simulink model "TF_simulink"  (R2025a)
settings: Solver=VariableStepAuto  StartTime=0.0  StopTime=50  RelTol=1e-3
undefined symbols (not defined in the file): b, bd, J, Jd, Jmotor, k, kd, ksea
libraries: slpidlib x2
settings Model: Creator=oskar  LastModifiedBy=oskar

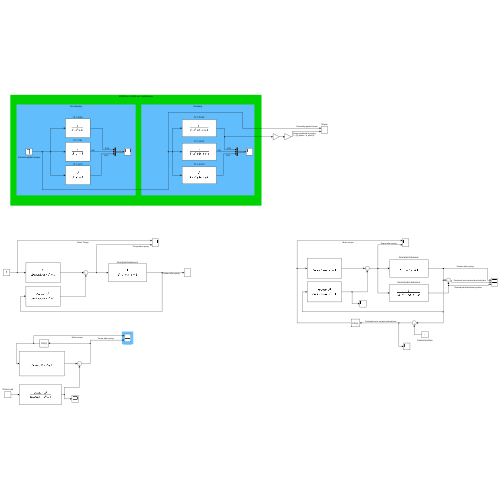
[thumbnail: Simulink's stored preview of the top-level diagram]
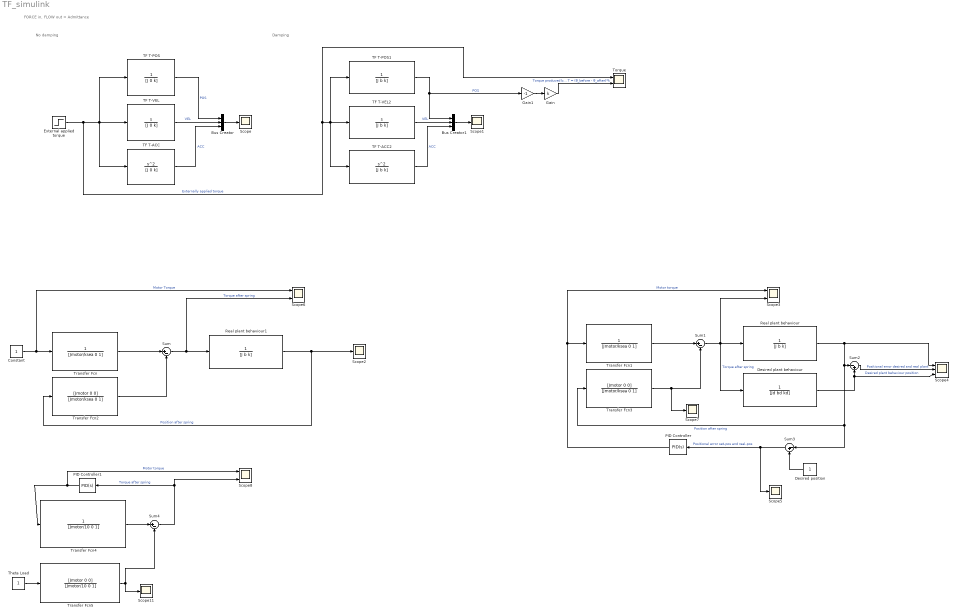
== system TF_simulink ==
  note: FORCE in, FLOW out = Admittance
  note: No damping
  note: Damping
  Bus Creator : BusCreator  Inputs=3
  Bus Creator1 : BusCreator  Inputs=3
  Constant : Constant
  Desired plant behaviour : TransferFcn  Denominator=[Jd bd kd]
  Desired position : Constant
  External applied torque : Step  Time=30  Before=1  After=0  SampleTime=0
  Gain : Gain  Gain=k
  Gain1 : Gain  Gain=-1
  PID Controller : slpidlib/PID Controller  Controller=PID  Form=Parallel  TimeDomain=Continuous-time  UseExternalTs=off  SampleTime=-1  IntegratorMethod=Forward Euler  FilterMethod=Forward Euler  ControllerParametersSource=internal  P=5  I=2  UseKiTs=off  D=0.01  UseExternalDerivativeSource=off  N=100  UseFilter=on  TunerSelectOption=Transfer Function Based (PID Tuner App)  InitialConditionSource=internal  InitialConditionForIntegrator=0  InitialConditionForFilter=0  DifferentiatorICPrevScaledInput=0  ExternalReset=none  TrackingMode=off  Kt=1  LimitOutput=off  SatLimitsSource=internal  UpperSaturationLimit=inf  LowerSaturationLimit=-inf  LinearizeAsGain=on  AntiWindupMode=none  Kb=1  LimitIntegrator=off  UpperIntegratorSaturationLimit=inf  LowerIntegratorSaturationLimit=-inf  POutMin=[]  POutMax=[]  IOutMin=[]  IOutMax=[]  DOutMin=[]  DOutMax=[]  NOutMin=[]  NOutMax=[]  SumOutMin=[]  SumOutMax=[]  SaturationOutMin=[]  SaturationOutMax=[]  PParamMin=[]  PParamMax=[]  IParamMin=[]  IParamMax=[]  DParamMin=[]  DParamMax=[]  NParamMin=[]  NParamMax=[]  KbParamMin=[]  KbParamMax=[]  KtParamMin=[]  KtParamMax=[]  KbOutMin=[]  KbOutMax=[]  KtOutMin=[]  KtOutMax=[]  IntegratorOutMin=[]  IntegratorOutMax=[]  FilterOutMin=[]  FilterOutMax=[]  SumI1OutMin=[]  SumI1OutMax=[]  SumI2OutMin=[]  SumI2OutMax=[]  SumI3OutMin=[]  SumI3OutMax=[]  SumI4OutMin=[]  SumI4OutMax=[]  SumDOutMin=[]  SumDOutMax=[]  DifferentiatorOutMin=[]  DifferentiatorOutMax=[]  FilterDiffOutCoefMin=[]  FilterDiffOutCoefMax=[]  ReciprocalOutMin=[]  ReciprocalOutMax=[]  SumDenOutMin=[]  SumDenOutMax=[]  SumNumOutMin=[]  SumNumOutMax=[]  DivideOutMin=[]  DivideOutMax=[]  UdiffTsProdOutMin=[]  UdiffTsProdOutMax=[]  NTsProdOutMin=[]  NTsProdOutMax=[]  UintegralTsProdOutMin=[]  UintegralTsProdOutMax=[]  UngainTsProdOutMin=[]  UngainTsProdOutMax=[]  ClampingZeroOutDataTypeStr=Inherit: Inherit via back propagation  ClampingZeroOutMin=[]  ClampingZeroOutMax=[]  FilterDenConstantOutDataTypeStr=Inherit: Inherit via back propagation  FilterDenConstantOutMin=[]  FilterDenConstantOutMax=[]  PCopyOutDataTypeStr=Inherit: Inherit via back propagation  PCopyOutMin=[]  PCopyOutMax=[]  NCopyOutDataTypeStr=Inherit: Inherit via back propagation  NCopyOutMin=[]  NCopyOutMax=[]  IntegratorContinuousStateAttributes=''  IntegratorStateMustResolveToSignalObject=off  IntegratorRTWStateStorageClass=Auto  FilterContinuousStateAttributes=''  FilterStateMustResolveToSignalObject=off  FilterRTWStateStorageClass=Auto  ParallelPVariant=InternalParameters  IdealPVariant=Disabled  IVariant=InternalParameters  DVariant=InternalParameters  IntegratorVariant=Continuous  SatVariant=Disabled  AWVariant=Passthrough  PCopyVariant=Disabled  TRVariant=Disabled  FdbkBlocksVariant=Forward  IdealPFdbkVariant=Disabled  SatFdbkVariant=Disabled  DerivativeFilterVariant=ContFilter  NVariant=InternalParameters  NCopyVariant=Disabled  FilterICVariant=InternalICsFilter  IntegratorICVariant=InternalICs  ExternalResetVariant=Disabled  TRSumVariant=Passthrough  SumFdbkVariant=Disabled  SumVariant=Sum_PID  TsampFilterVariant=InternalTs  TsampNgainVariant=Passthrough  TsampIntegralVariant=Disabled_SignalSpec  ExternalSaturationOutDataTypeStr=Inherit: Same as second input  DerivativeSourceVariant=ErrorSignal  PreIntVariant=InternalPreInt
  PID Controller1 : slpidlib/PID Controller  Controller=PID  Form=Parallel  TimeDomain=Continuous-time  UseExternalTs=off  SampleTime=-1  IntegratorMethod=Forward Euler  FilterMethod=Forward Euler  ControllerParametersSource=internal  P=10  I=0  UseKiTs=off  D=0  UseExternalDerivativeSource=off  N=100  UseFilter=on  TunerSelectOption=Transfer Function Based (PID Tuner App)  InitialConditionSource=internal  InitialConditionForIntegrator=0  InitialConditionForFilter=0  DifferentiatorICPrevScaledInput=0  ExternalReset=none  TrackingMode=off  Kt=1  LimitOutput=off  SatLimitsSource=internal  UpperSaturationLimit=inf  LowerSaturationLimit=-inf  LinearizeAsGain=on  AntiWindupMode=none  Kb=1  LimitIntegrator=off  UpperIntegratorSaturationLimit=inf  LowerIntegratorSaturationLimit=-inf  POutMin=[]  POutMax=[]  IOutMin=[]  IOutMax=[]  DOutMin=[]  DOutMax=[]  NOutMin=[]  NOutMax=[]  SumOutMin=[]  SumOutMax=[]  SaturationOutMin=[]  SaturationOutMax=[]  PParamMin=[]  PParamMax=[]  IParamMin=[]  IParamMax=[]  DParamMin=[]  DParamMax=[]  NParamMin=[]  NParamMax=[]  KbParamMin=[]  KbParamMax=[]  KtParamMin=[]  KtParamMax=[]  KbOutMin=[]  KbOutMax=[]  KtOutMin=[]  KtOutMax=[]  IntegratorOutMin=[]  IntegratorOutMax=[]  FilterOutMin=[]  FilterOutMax=[]  SumI1OutMin=[]  SumI1OutMax=[]  SumI2OutMin=[]  SumI2OutMax=[]  SumI3OutMin=[]  SumI3OutMax=[]  SumI4OutMin=[]  SumI4OutMax=[]  SumDOutMin=[]  SumDOutMax=[]  DifferentiatorOutMin=[]  DifferentiatorOutMax=[]  FilterDiffOutCoefMin=[]  FilterDiffOutCoefMax=[]  ReciprocalOutMin=[]  ReciprocalOutMax=[]  SumDenOutMin=[]  SumDenOutMax=[]  SumNumOutMin=[]  SumNumOutMax=[]  DivideOutMin=[]  DivideOutMax=[]  UdiffTsProdOutMin=[]  UdiffTsProdOutMax=[]  NTsProdOutMin=[]  NTsProdOutMax=[]  UintegralTsProdOutMin=[]  UintegralTsProdOutMax=[]  UngainTsProdOutMin=[]  UngainTsProdOutMax=[]  ClampingZeroOutDataTypeStr=Inherit: Inherit via back propagation  ClampingZeroOutMin=[]  ClampingZeroOutMax=[]  FilterDenConstantOutDataTypeStr=Inherit: Inherit via back propagation  FilterDenConstantOutMin=[]  FilterDenConstantOutMax=[]  PCopyOutDataTypeStr=Inherit: Inherit via back propagation  PCopyOutMin=[]  PCopyOutMax=[]  NCopyOutDataTypeStr=Inherit: Inherit via back propagation  NCopyOutMin=[]  NCopyOutMax=[]  IntegratorContinuousStateAttributes=''  IntegratorStateMustResolveToSignalObject=off  IntegratorRTWStateStorageClass=Auto  FilterContinuousStateAttributes=''  FilterStateMustResolveToSignalObject=off  FilterRTWStateStorageClass=Auto  ParallelPVariant=InternalParameters  IdealPVariant=Disabled  IVariant=InternalParameters  DVariant=InternalParameters  IntegratorVariant=Continuous  SatVariant=Disabled  AWVariant=Passthrough  PCopyVariant=Disabled  TRVariant=Disabled  FdbkBlocksVariant=Forward  IdealPFdbkVariant=Disabled  SatFdbkVariant=Disabled  DerivativeFilterVariant=ContFilter  NVariant=InternalParameters  NCopyVariant=Disabled  FilterICVariant=InternalICsFilter  IntegratorICVariant=InternalICs  ExternalResetVariant=Disabled  TRSumVariant=Passthrough  SumFdbkVariant=Disabled  SumVariant=Sum_PID  TsampFilterVariant=InternalTs  TsampNgainVariant=Passthrough  TsampIntegralVariant=Disabled_SignalSpec  ExternalSaturationOutDataTypeStr=Inherit: Same as second input  DerivativeSourceVariant=ErrorSignal  PreIntVariant=InternalPreInt
  Real plant behaviour : TransferFcn  Denominator=[J b k]
  Real plant behaviour1 : TransferFcn  Denominator=[J b k]
  Scope{,1..2,5,7,11} (6 alike) : Scope
      Scope settings: ActiveDisplayYMinimum=-4.4747944880610575  ActiveDisplayYMaximum=4.4748865420859838
      Scope1 settings: ActiveDisplayYMinimum=-0.19190828565154572  ActiveDisplayYMaximum=0.31988040805006046
      Scope11 settings: ActiveDisplayYMinimum=-12.499943965538082  ActiveDisplayYMaximum=12.499993773948676  DataLoggingVariableName=ScopeData10
      Scope2 settings: ActiveDisplayYMinimum=-0.013105853522271727  ActiveDisplayYMaximum=0.11795268170044557  DataLoggingVariableName=ScopeData3
      Scope5 settings: ActiveDisplayYMinimum=-0.1242629467640454  ActiveDisplayYMaximum=1.1249181051960051  DataLoggingVariableName=ScopeData6
      Scope7 settings: ActiveDisplayYMinimum=-1  ActiveDisplayYMaximum=1  DataLoggingVariableName=ScopeData8
  Scope3 : Scope  NumInputPorts=2
      settings: ActiveDisplayYMinimum=-1.2492300800290874  ActiveDisplayYMaximum=11.243070720261789  DataLoggingVariableName=ScopeData4
  Scope4 : Scope  NumInputPorts=3
      settings: ActiveDisplayYMinimum=-0.24983177276775023  ActiveDisplayYMaximum=2.2484859549097527  DataLoggingVariableName=ScopeData5
  Scope6 : Scope  NumInputPorts=2
      settings: ActiveDisplayYMinimum=-0.64476081445685562  ActiveDisplayYMaximum=1.6782502736646918  DataLoggingVariableName=ScopeData7
  Scope8 : Scope  NumInputPorts=2
      settings: ActiveDisplayYMinimum=-1.2146071971742971E+293  ActiveDisplayYMaximum=1.3495635524158854E+292  DataLoggingVariableName=ScopeData11
  Sum : Sum  Inputs=|+-
  Sum1 : Sum  Inputs=|+-
  Sum2 : Sum  Inputs=|-+
  Sum3 : Sum  Inputs=|-+
  Sum4 : Sum  Inputs=|+-
  TF T-ACC : TransferFcn  Numerator=[1 0 0]  Denominator=[J 0 k]
  TF T-ACC2 : TransferFcn  Numerator=[1 0 0]  Denominator=[J b k]
  TF T-POS : TransferFcn  Denominator=[J 0 k]
  TF T-POS1 : TransferFcn  Denominator=[J b k]
  TF T-VEL : TransferFcn  Numerator=[1 0]  Denominator=[J 0 k]
  TF T-VEL2 : TransferFcn  Numerator=[1 0]  Denominator=[J b k]
  Theta Load : Constant
  Torque : Scope  NumInputPorts=2
      settings: ActiveDisplayYMinimum=-1.2499999999999998  ActiveDisplayYMaximum=1.25  DataLoggingVariableName=ScopeData2
  Transfer Fcn : TransferFcn  Denominator=[Jmotor/ksea 0 1]
  Transfer Fcn1 : TransferFcn  Denominator=[Jmotor/ksea 0 1]
  Transfer Fcn2 : TransferFcn  Numerator=[Jmotor 0 0]  Denominator=[Jmotor/ksea 0 1]
  Transfer Fcn3 : TransferFcn  Numerator=[Jmotor 0 0]  Denominator=[Jmotor/ksea 0 1]
  Transfer Fcn4 : TransferFcn  Denominator=[Jmotor/10 0 1]
  Transfer Fcn5 : TransferFcn  Numerator=[Jmotor 0 0]  Denominator=[Jmotor/10 0 1]
  wires:
  TF T-POS/1 -> Bus Creator/1  "POS"
  TF T-VEL/1 -> Bus Creator/2  "VEL"
  TF T-ACC/1 -> Bus Creator/3  "ACC"
  Bus Creator/1 -> Scope/1
  Bus Creator1/1 -> Scope1/1
  TF T-POS1/1 -> Gain1/1, Bus Creator1/1  "POS"
  TF T-ACC2/1 -> Bus Creator1/3  "ACC"
  External applied torque/1 -> Torque/1, TF T-ACC2/1, TF T-VEL2/1, TF T-POS1/1, TF T-VEL/1, TF T-POS/1, TF T-ACC/1  "Externally applied torque"
  TF T-VEL2/1 -> Bus Creator1/2  "VEL"
  Gain/1 -> Torque/2  "Torque produced by spring T = (θ_before - θ_after)*k"
  Gain1/1 -> Gain/1
  Transfer Fcn/1 -> Sum/1
  Transfer Fcn2/1 -> Sum/2
  Sum/1 -> Scope6/2, Real plant behaviour1/1  "Torque after spring"
  Real plant behaviour1/1 -> Transfer Fcn2/1, Scope2/1  "Position after spring"
  Real plant behaviour/1 -> Scope4/1, Sum2/1, Sum3/1, Transfer Fcn3/1  "Position after spring"
  Transfer Fcn3/1 -> Scope7/1, Sum1/2
  Sum1/1 -> Desired plant behaviour/1, Scope3/2, Real plant behaviour/1  "Torque after spring"
  Transfer Fcn1/1 -> Sum1/1
  Desired plant behaviour/1 -> Scope4/3, Sum2/2  "Desired plant behaviour position"
  Sum2/1 -> Scope4/2  "Positional error desired and real plant"
  Desired position/1 -> Sum3/2
  Sum3/1 -> Scope5/1, PID Controller/1  "Positional error set-pos and real-pos"
  PID Controller/1 -> Transfer Fcn1/1, Scope3/1  "Motor torque"
  Constant/1 -> Transfer Fcn/1, Scope6/1  "Motor Torque"
  Transfer Fcn4/1 -> Sum4/1
  Sum4/1 -> PID Controller1/1, Scope8/2  "Torque after spring"
  Transfer Fcn5/1 -> Sum4/2, Scope11/1
  Theta Load/1 -> Transfer Fcn5/1
  PID Controller1/1 -> Scope8/1, Transfer Fcn4/1  "Motor torque"
